simulink model "sl_ros_params"  (R2015b)
settings: Solver=VariableStepAuto  StartTime=0.0  StopTime=inf  RelTol=1e-3
libraries: robotlib x4
settings Model: Creator=zihan  LastModifiedBy=zihan

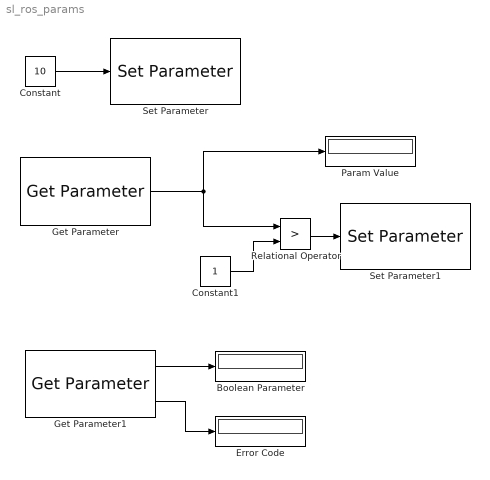
== system sl_ros_params ==
  Boolean Parameter : Display
  Constant : Constant  Value=10
  Constant1 : Constant
  Error Code : Display
  Get Parameter : robotlib/Get Parameter  SourceLibraryInfo=This block requires Robotics System Toolbox  ParameterSource=Specify your own  ParameterName=/my_int  ParameterType=double  ParameterInitialValue=0.0  SampleTime=-1  ShowErrorCodeOutput=off  ModelName=sl_ros_params  BlockId=ParamGet_sl_ros_params_3
  Get Parameter1 : robotlib/Get Parameter  SourceLibraryInfo=This block requires Robotics System Toolbox  ParameterSource=Select from ROS network  ParameterName=/my_boolean  ParameterType=boolean  ParameterInitialValue=0.0  SampleTime=-1  ShowErrorCodeOutput=on  ModelName=sl_ros_params  BlockId=ParamGet_sl_ros_params_8
  Param Value : Display
  Relational Operator : RelationalOperator  Operator=>  OutDataTypeStr=boolean
  Set Parameter : robotlib/Set Parameter  SourceLibraryInfo=This block requires Robotics System Toolbox  ParameterSource=Specify your own  ParameterName=/my_int  ParameterType=double  ModelName=sl_ros_params  BlockId=ParamSet_sl_ros_params_2
  Set Parameter1 : robotlib/Set Parameter  SourceLibraryInfo=This block requires Robotics System Toolbox  ParameterSource=Specify your own  ParameterName=/my_boolean  ParameterType=boolean  ModelName=sl_ros_params  BlockId=ParamSet_sl_ros_params_7
  wires:
  Constant/1 -> Set Parameter/1
  Get Parameter/1 -> Relational Operator/1, Param Value/1
  Constant1/1 -> Relational Operator/2
  Relational Operator/1 -> Set Parameter1/1
  Get Parameter1/1 -> Boolean Parameter/1
  Get Parameter1/2 -> Error Code/1
